simulink model "A3_MPC"  (R2012b)
settings: Solver=ode45  StartTime=0.0  StopTime=100  RelTol=1e-3
PreLoadFcn:
  | Initialize
StopFcn:
  | A3_plot_and_save
undefined symbols (not defined in the file or in its folder): control, heights, P, PlotTanks2
libraries: simulink x4
settings Model: Creator=tsladeche  LastModifiedBy=John
settings DataIOCC: SignalLoggingSaveFormat=ModelDataLogs
settings DebuggingCC: FcnCallInpInsideContextMsg=UseLocalSettings  StrictBusMsg=Warning
settings GRTTargetCC: CombineOutputUpdateFcns=off  GRTInterface=on

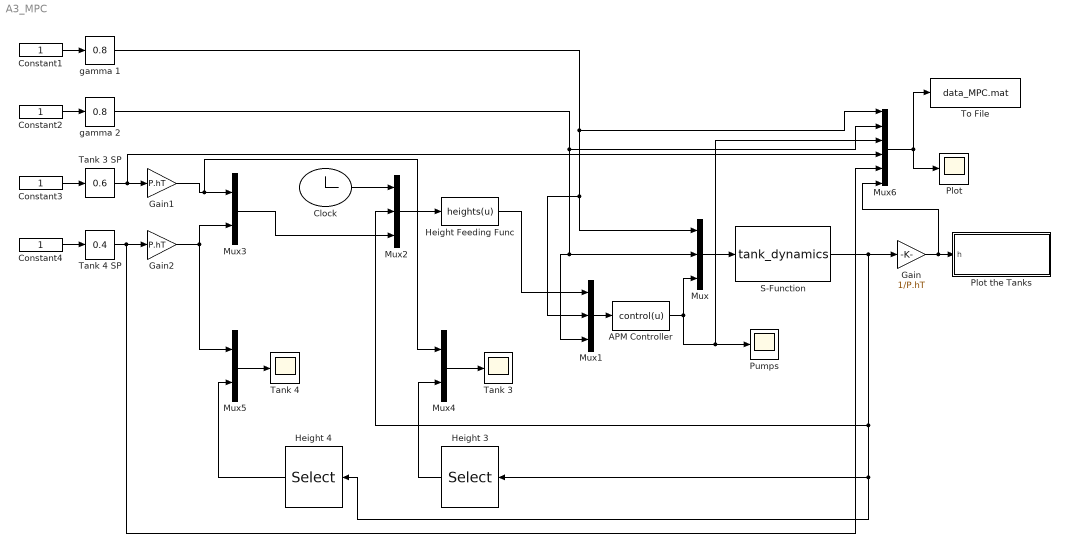
== system A3_MPC ==
  APM Controller : MATLABFcn  MATLABFcn=control(u)  OutputDimensions=2  SampleTime=.5
  Clock : Clock
  Constant{1..4} (4 alike) : Constant
  Gain : Gain  Gain=1/P.hT
  Gain1 : Gain  Gain=P.hT
  Gain2 : Gain  Gain=P.hT
  Height 3 : Selector  InputPortWidth=4  IndexOptions=Index vector (dialog)  Indices=3  OutputSizes=1
  Height 4 : Selector  InputPortWidth=4  IndexOptions=Index vector (dialog)  Indices=4  OutputSizes=1
  Height Feeding Func : MATLABFcn  MATLABFcn=heights(u)  OutputDimensions=6  SampleTime=.5
  Mux : Mux  Inputs=3
  Mux1 : Mux  Inputs=3
  Mux2 : Mux  Inputs=3
  Mux3 : Mux  Inputs=2
  Mux4 : Mux  Inputs=2
  Mux5 : Mux  Inputs=2
  Mux6 : Mux  Inputs=6
  Plot : Scope
      settings: YMin=0.1  YMax=1
  Plot the Tanks : Subsystem
  Pumps : Scope
      settings: YMin=5.55112e-17  YMax=1
  S-Function : S-Function  FunctionName=tank_dynamics  Parameters=P  EnableBusSupport=off
  Tank 3 : Scope
      settings: TimeRange=100  YMin=15  YMax=29  SaveName=ScopeData2
  Tank 3 SP : simulink/Math Operations/Slider Gain  low=0  gain=0.6  high=1
  Tank 4 : Scope
      settings: TimeRange=100  YMin=15  YMax=29  SaveName=ScopeData3
  Tank 4 SP : simulink/Math Operations/Slider Gain  low=0  gain=0.4  high=1
  To File : ToFile  Filename=data_MPC.mat  MatrixName=tanks  SampleTime=1
  gamma 1 : simulink/Math Operations/Slider Gain  low=0  gain=0.8  high=1
  gamma 2 : simulink/Math Operations/Slider Gain  low=0  gain=0.8  high=1
  wires:
  Constant2/1 -> gamma 2/1
  Constant1/1 -> gamma 1/1
  gamma 1/1 -> Mux6/1, Mux/1, Mux1/2
  gamma 2/1 -> Mux6/2, Mux/2, Mux1/3
  APM Controller/1 -> Mux6/3, Pumps/1, Mux/3
  Mux1/1 -> APM Controller/1
  Height Feeding Func/1 -> Mux1/1
  Mux2/1 -> Height Feeding Func/1
  Clock/1 -> Mux2/1
  Gain/1 -> Mux6/6, Plot the Tanks/1(h)
  S-Function/1 -> Gain/1, Height 4/1, Height 3/1, Mux2/2
  Mux/1 -> S-Function/1
  Constant3/1 -> Tank 3 SP/1
  Constant4/1 -> Tank 4 SP/1
  Tank 4 SP/1 -> Mux6/5, Gain2/1
  Tank 3 SP/1 -> Mux6/4, Gain1/1
  Gain2/1 -> Mux3/2, Mux5/1
  Gain1/1 -> Mux3/1, Mux4/1
  Mux3/1 -> Mux2/3
  Height 3/1 -> Mux4/2
  Height 4/1 -> Mux5/2
  Mux5/1 -> Tank 4/1
  Mux4/1 -> Tank 3/1
  Mux6/1 -> To File/1, Plot/1

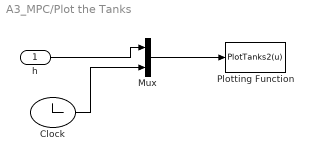
== system A3_MPC/Plot the Tanks ==
  h : Inport
  Clock : Clock
  Mux : Mux  Inputs=2
  Plotting Function : MATLABFcn  MATLABFcn=PlotTanks2(u)  OutputDimensions=0  SampleTime=1.0
  wires:
  Mux/1 -> Plotting Function/1
  Clock/1 -> Mux/2
  h/1 -> Mux/1
